simulink model "phase_attack"  (R2021a)
settings: Solver=ode23t  StartTime=0.0  StopTime=10.0  RelTol=1e-3
libraries: spsPowerPhasorLib x2
settings Model: Creator=Suman  LastModifiedBy=Suman

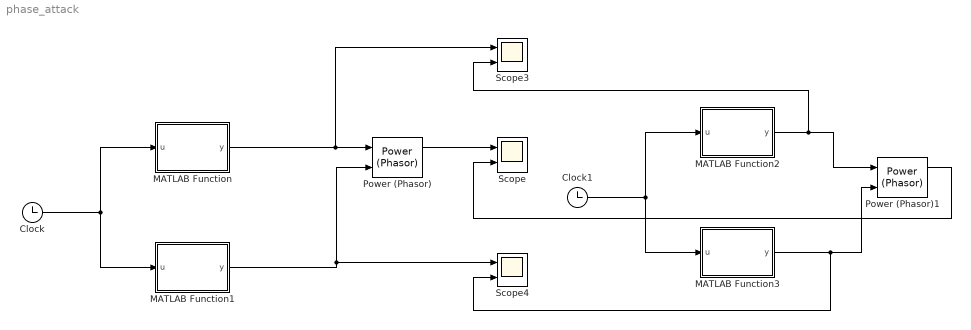
== system phase_attack ==
  Clock : Clock
  Clock1 : Clock
  MATLAB Function : MATLAB Function  TreatAsAtomicUnit=on
  MATLAB Function1 : MATLAB Function  TreatAsAtomicUnit=on
  MATLAB Function2 : MATLAB Function  TreatAsAtomicUnit=on
  MATLAB Function3 : MATLAB Function  TreatAsAtomicUnit=on
  Power (Phasor) : spsPowerPhasorLib/Power (Phasor)
      settings: SourceProductBaseCode=PS
  Power (Phasor)1 : spsPowerPhasorLib/Power (Phasor)
      settings: SourceProductBaseCode=PS
  Scope : Scope  NumInputPorts=2
  Scope3 : Scope  NumInputPorts=2
  Scope4 : Scope  NumInputPorts=2
  wires:
  Clock/1 -> MATLAB Function1/1(u), MATLAB Function/1(u)
  MATLAB Function/1(y) -> Scope3/1, Power (Phasor)/1
  MATLAB Function1/1(y) -> Scope4/1, Power (Phasor)/2
  MATLAB Function3/1(y) -> Scope4/2, Power (Phasor)1/2
  MATLAB Function2/1(y) -> Scope3/2, Power (Phasor)1/1
  Clock1/1 -> MATLAB Function2/1(u), MATLAB Function3/1(u)
  Power (Phasor)/1 -> Scope/1
  Power (Phasor)1/1 -> Scope/2

== matlab function phase_attack/MATLAB Function ==
  data: u input; y output
function y = fcn(u)

y =sin(u);

== matlab function phase_attack/MATLAB Function2 ==
  data: u input; y output
function y = fcn(u)

y =sin(u+pi/4);

== matlab function phase_attack/MATLAB Function3 ==
  data: u input; y output
function y = fcn(u)

y = cos(u+pi/4);

== matlab function phase_attack/MATLAB Function1 ==
  data: u input; y output
function y = fcn(u)

y = cos(u);
